simulink model "UART"  (R2026a)
settings: Solver=FixedStepDiscrete  StopTime=12/9600  FixedStep=1/9600
libraries: simulink x3

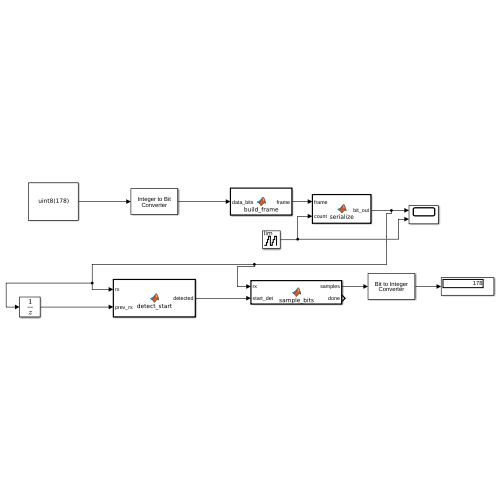
[thumbnail: Simulink's stored preview of the top-level diagram]
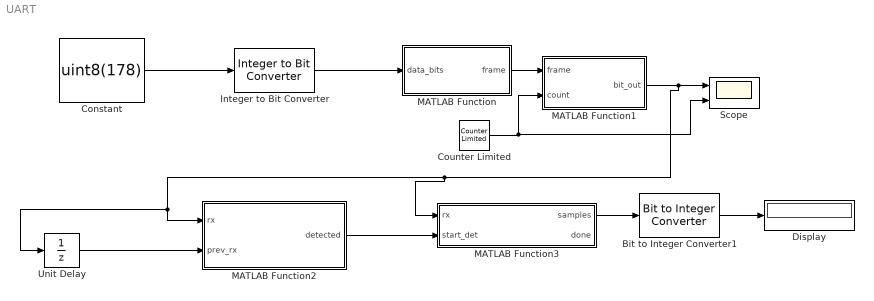
== system UART ==
  Bit to Integer Converter1 : simulink/Logic and Bit Operations/Bit to Integer Converter  nbits=8  bitOrder=MSB first  signedOutputValues=Unsigned  outDtype=Inherit via internal rule  outDtypeSigned=Inherit via internal rule
  Constant : Constant  Value=uint8(178)
  Counter Limited : simulink/Sources/Counter Limited  uplimit=9  tsamp=-1
  Display : Display
  Integer to Bit Converter : simulink/Logic and Bit Operations/Integer to Bit Converter  nbits=8  signedInputValues=Unsigned  bitOrder=MSB first  outDtype=Inherit via internal rule
  MATLAB Function : MATLAB Function  TreatAsAtomicUnit=on
  MATLAB Function1 : MATLAB Function  TreatAsAtomicUnit=on
  MATLAB Function2 : MATLAB Function  TreatAsAtomicUnit=on
  MATLAB Function3 : MATLAB Function  TreatAsAtomicUnit=on
  Scope : Scope  NumInputPorts=2
      settings: ActiveDisplayYMinimum=-2.7754053661281493  ActiveDisplayYMaximum=11.586834178285683
  Unit Delay : UnitDelay  InitialCondition=1  SampleTime=-1
  wires:
  Constant/1 -> Integer to Bit Converter/1
  Integer to Bit Converter/1 -> MATLAB Function/1(data_bits)
  MATLAB Function/1(frame) -> MATLAB Function1/1(frame)
  MATLAB Function1/1(bit_out) -> MATLAB Function2/1(rx), Unit Delay/1, MATLAB Function3/1(rx), Scope/1
  Counter Limited/1 -> Scope/2, MATLAB Function1/2(count)
  Unit Delay/1 -> MATLAB Function2/2(prev_rx)
  MATLAB Function2/1(detected) -> MATLAB Function3/2(start_det)
  MATLAB Function3/1(samples) -> Bit to Integer Converter1/1
  Bit to Integer Converter1/1 -> Display/1

== matlab function UART/MATLAB Function ==
  data: data_bits input; frame output
function frame = build_frame(data_bits)
start_bit = double(0);
stop_bit  = double(1);
frame = [start_bit; double(data_bits); stop_bit];
end

== matlab function UART/MATLAB Function2 ==
  data: rx input; detected output; prev_rx input

function detected = detect_start(rx, prev_rx)
   detected = uint8((prev_rx == 1) && (rx == 0));
end

== matlab function UART/MATLAB Function3 ==
  data: rx input; samples output; start_det input; done output
function [samples, done] = sample_bits(rx, start_det)
persistent bit_count sample_buf active skip

if isempty(active)
    active = false;
    bit_count = int32(0);
    sample_buf = zeros(8,1,'double');
    skip = false;
end

samples = sample_buf;
done = double(0);

if start_det == 1 && ~active
    active = true;
    bit_count = int32(0);
    skip = true;
end

if active
    if skip
        skip = false;
    elseif bit_count < int32(8)
        bit_count = bit_count + int32(1);
        sample_buf(bit_count) = double(rx);

        if bit_count == int32(8)
            samples = sample_buf;
            done = double(1);
            active = false;
            bit_count = int32(0);
        end
    end
end
end

== matlab function UART/MATLAB Function1 ==
  data: frame input; bit_out output; count input

   function bit_out = serialize(frame, count)
  idx = mod(int32(count), int32(10)) + int32(1);
  bit_out = double(frame(idx));
end
